simulink model "EulerPIDJoint_Copy"  (Simulink 7.6)
settings: Solver=ode3  StartTime=0.0  StopTime=8  FixedStep=Ts  RelTol=1e-3
InitFcn:
  | eval('Config');
  | eval('RobotCtlCfg');
values from neighbouring files (symbols this model uses):
  a2 = 0    [Config.m]    (also in CtrPlatformCfg.m)
  a3 = 0    [Config.m]    (also in CtrPlatformCfg.m)
  a4 = 0    [Config.m]    (also in CtrPlatformCfg.m)
  a5 = 90    [Config.m]    (also in CtrPlatformCfg.m)
  a6 = 0    [Config.m]    (also in CtrPlatformCfg.m)
  Cen_EU = Cen    [DynEulerTest.m]
  DH_EU = [266     300     0       0       1016     0      174 ... (first row only)    [DynEulerTest.m]
  freq = tvel/radius    (= 1)    [Config.m]    (also in CtrPlatformCfg.m)
  Ft_EU = [0;0;0;0;0;0]    [DynEulerTest.m]
  Gravity = 9.8    [Config.m]    (also in CtrPlatformCfg.m)
  Ie_EU = [Ie1;Ie2;Ie3;Ie4;Ie5;Ie6]    [DynEulerTest.m]
  in1 = [5.2954 -0.2565 -0.6366;-0.2565 4.7000 0.2830;-0.6366 0.2829 5.8635]    [Config.m]    (also in CtrPlatformCfg.m; DynEulerTest.m; EfDynCAD.m = [0.54  -0.01 0.23)
  in2 = [5.8840 0.0072 0.0135;0.0072 6.0178 -0.1907;0.0135 -0.1907 0.3374]    [Config.m]    (also in CtrPlatformCfg.m; DynEulerTest.m; EfDynCAD.m = (R_x*R_z)*in2*(R_x*R_z)')
  in3 = [1.8201 -0.2274 -0.3112;-0.2274 2.2537 -0.1441;-0.3112 -0.1441 1.9485]    [Config.m]    (also in CtrPlatformCfg.m; DynEulerTest.m; EfDynCAD.m = (R_x*R_z)*in3*(R_x*R_z)')
  in4 = [0.0607 -0.0922 0;-0.0922 1.4493 0;0 0 1.4620]    [Config.m]    (also in CtrPlatformCfg.m; DynEulerTest.m = [0.0607 -0.0922 0;-0.0922 1.4493 0;0 0,1.4620]; EfDynCAD.m = (R_y*Rz)*in4*(R_y*Rz)')
  in5 = [0.0191 0.0032 0;0.0032 0.0228 0;0 0 0.0291]    [Config.m]    (also in CtrPlatformCfg.m; DynEulerTest.m; EfDynCAD.m = (R_x*R_y)*in5*(R_x*R_y)')
  in6 = [0.0012 0 0;0 0.0007 0;0 0 0.0007]    [Config.m]    (also in CtrPlatformCfg.m; DynEulerTest.m; EfDynCAD.m = (R_y*Rz)*in6*(R_y*Rz)')
  init_Endx = gd_init(1,4)    [Config.m]    (also in CtrPlatformCfg.m)
  init_Endy = gd_init(2,4)    [Config.m]    (also in CtrPlatformCfg.m)
  init_Endz = gd_init(3,4)    [Config.m]    (also in CtrPlatformCfg.m)
  init_Rot = gd_init(1:3,1:3)    [Config.m]    (also in CtrPlatformCfg.m)
  L = [l1 l2 l3 l4 l5 l6 l7 l8 l9]    [Config.m]    (also in CtrPlatformCfg.m)
  ma1 = 170.31    [Config.m]    (also in CtrPlatformCfg.m; DynEulerTest.m; EfDynCAD.m = 77.75)
  ma2 = 63.74    [Config.m]    (also in CtrPlatformCfg.m; DynEulerTest.m; EfDynCAD.m = 32.31)
  ma3 = 98.98    [Config.m]    (also in CtrPlatformCfg.m; DynEulerTest.m; EfDynCAD.m = 18.61)
  ma4 = 24.46    [Config.m]    (also in CtrPlatformCfg.m; DynEulerTest.m; EfDynCAD.m = 15.65)
  ma5 = 5.24    [Config.m]    (also in CtrPlatformCfg.m; DynEulerTest.m; EfDynCAD.m = 3.32)
  ma6 = 0.6    [Config.m]    (also in CtrPlatformCfg.m; DynEulerTest.m; EfDynCAD.m)
  Ma_EU = Ma    [DynEulerTest.m]
  Rad2Line = Gear*EncRes/(2*pi)    [Config.m]    (also in CtrPlatformCfg.m)
  Ts = 1/FrHz    (= 0.00025)    [Config.m]    (also in CtrPlatformCfg.m)
  tvel = 120    [Config.m]    (also in CtrPlatformCfg.m)
undefined symbols (not defined in the file or in its folder): a1, DiscIntNeverNeededParam, jointAugKp, jointAugKv, PRBSGain, PRBSOffset, PRBSTimeLength, PulseFrq, PulseGain, RobotAxis, SineFrq, SineGain, V2T
libraries: simulink x58, mblibv1 x41, powerlib_extras x7
(part 4 of 5)

== system EulerPIDJoint_Copy/Display/GeneralAccDisplay/Jnt3/Display ==
  GeneralAcc3 : Inport
  Ref_GeneralAcc3 : Inport  Port=2
  AVx : Scope  NumInputPorts=2
      settings: TimeRange=10  YMin=-2.999999999999999e-017~-1  YMax=4e-017~1
  "AVy " : Scope  NumInputPorts=2
      settings: YMin=-5~-5  YMax=5~5
  AVz : Scope  NumInputPorts=2
      settings: YMin=-5~-5  YMax=5~5  SaveName=ScopeData2
  AWx : Scope  NumInputPorts=2
      settings: YMin=-5~-5  YMax=5~5  SaveName=ScopeData3
  AWy : Scope  NumInputPorts=2
      settings: TimeRange=10  YMin=-4.18~4.060000000000001  YMax=-4.04~4.2  SaveName=ScopeData4
  AWz : Scope  NumInputPorts=2
      settings: TimeRange=10  YMin=-1.6e-006~-0.003  YMax=4e-007~0.004  SaveName=ScopeData5
  Demux : Demux  Outputs=6
  Demux1 : Demux  Outputs=6
  "Encoder " : ToWorkspace  VariableName=EncGenAccJ3  SampleTime=-1  SaveFormat=Structure
  Err{1..6} (6 alike) : Scope
      Err1 settings: SaveName=ScopeData6
      Err2 settings: SaveName=ScopeData7
      Err3 settings: SaveName=ScopeData8
      Err4 settings: SaveName=ScopeData9
      Err5 settings: TimeRange=3  YMin=-2.5  YMax=1  SaveName=ScopeData10
      Err6 settings: SaveName=ScopeData11
  "Ref " : ToWorkspace  VariableName=RefGenAccJ3  SampleTime=-1  SaveFormat=Structure
  Sum{,1..5} (6 alike) : Sum  Inputs=+|-
  wires:
  Demux1/6 -> Sum5/2, AWz/2
  Demux1/5 -> Sum4/2, AWy/2
  Demux1/4 -> AWx/2, Sum3/2
  Demux1/3 -> Sum2/2, AVz/2
  Demux1/2 -> Sum1/2, "AVy "/2
  Demux/6 -> Sum5/1, AWz/1
  Demux/5 -> Sum4/1, AWy/1
  Demux/4 -> AWx/1, Sum3/1
  Demux/3 -> Sum2/1, AVz/1
  Demux/2 -> Sum1/1, "AVy "/1
  Demux1/1 -> AVx/2, Sum/2
  Demux/1 -> AVx/1, Sum/1
  Ref_GeneralAcc3/1 -> "Ref "/1, Demux1/1
  GeneralAcc3/1 -> "Encoder "/1, Demux/1
  Sum5/1 -> Err6/1
  Sum4/1 -> Err5/1
  Sum3/1 -> Err4/1
  Sum2/1 -> Err3/1
  Sum1/1 -> Err2/1
  Sum/1 -> Err1/1

== system EulerPIDJoint_Copy/Display/GeneralAccDisplay/Jnt4/Display ==
  GeneralAcc4 : Inport
  Ref_GeneralAcc4 : Inport  Port=2
  AVx : Scope  NumInputPorts=2
      settings: TimeRange=10  YMin=-2.999999999999999e-017~-1  YMax=4e-017~1
  "AVy " : Scope  NumInputPorts=2
      settings: YMin=-5~-5  YMax=5~5
  AVz : Scope  NumInputPorts=2
      settings: YMin=-5~-5  YMax=5~5  SaveName=ScopeData2
  AWx : Scope  NumInputPorts=2
      settings: YMin=-5~-5  YMax=5~5  SaveName=ScopeData3
  AWy : Scope  NumInputPorts=2
      settings: TimeRange=10  YMin=-4.18~4.060000000000001  YMax=-4.04~4.2  SaveName=ScopeData4
  AWz : Scope  NumInputPorts=2
      settings: TimeRange=10  YMin=-1.6e-006~-0.003  YMax=4e-007~0.004  SaveName=ScopeData5
  Demux : Demux  Outputs=6
  Demux1 : Demux  Outputs=6
  "Encoder " : ToWorkspace  VariableName=EncGenAccJ4  SampleTime=-1  SaveFormat=Structure
  Err{1..6} (6 alike) : Scope
      Err1 settings: SaveName=ScopeData6
      Err2 settings: SaveName=ScopeData7
      Err3 settings: SaveName=ScopeData8
      Err4 settings: SaveName=ScopeData9
      Err5 settings: TimeRange=3  YMin=-2.5  YMax=1  SaveName=ScopeData10
      Err6 settings: SaveName=ScopeData11
  "Ref " : ToWorkspace  VariableName=RefGenAccJ4  SampleTime=-1  SaveFormat=Structure
  Sum{,1..5} (6 alike) : Sum  Inputs=+|-
  wires:
  Sum/1 -> Err1/1
  Sum1/1 -> Err2/1
  Sum2/1 -> Err3/1
  Sum3/1 -> Err4/1
  Sum4/1 -> Err5/1
  Sum5/1 -> Err6/1
  GeneralAcc4/1 -> Demux/1, "Encoder "/1
  Ref_GeneralAcc4/1 -> Demux1/1, "Ref "/1
  Demux/1 -> Sum/1, AVx/1
  Demux1/1 -> Sum/2, AVx/2
  Demux/2 -> "AVy "/1, Sum1/1
  Demux/3 -> AVz/1, Sum2/1
  Demux/4 -> Sum3/1, AWx/1
  Demux/5 -> AWy/1, Sum4/1
  Demux/6 -> AWz/1, Sum5/1
  Demux1/2 -> "AVy "/2, Sum1/2
  Demux1/3 -> AVz/2, Sum2/2
  Demux1/4 -> Sum3/2, AWx/2
  Demux1/5 -> AWy/2, Sum4/2
  Demux1/6 -> AWz/2, Sum5/2

== system EulerPIDJoint_Copy/Display/GeneralAccDisplay/Jnt5/Display ==
  GeneralAcc5 : Inport
  Ref_GeneralAcc5 : Inport  Port=2
  AVx : Scope  NumInputPorts=2
      settings: TimeRange=10  YMin=-2.999999999999999e-017~-1  YMax=4e-017~1
  "AVy " : Scope  NumInputPorts=2
      settings: YMin=-5~-5  YMax=5~5
  AVz : Scope  NumInputPorts=2
      settings: YMin=-5~-5  YMax=5~5  SaveName=ScopeData2
  AWx : Scope  NumInputPorts=2
      settings: YMin=-5~-5  YMax=5~5  SaveName=ScopeData3
  AWy : Scope  NumInputPorts=2
      settings: TimeRange=10  YMin=-4.18~4.060000000000001  YMax=-4.04~4.2  SaveName=ScopeData4
  AWz : Scope  NumInputPorts=2
      settings: TimeRange=10  YMin=-1.6e-006~-0.003  YMax=4e-007~0.004  SaveName=ScopeData5
  Demux : Demux  Outputs=6
  Demux1 : Demux  Outputs=6
  "Encoder " : ToWorkspace  VariableName=EncGenAccJ5  SampleTime=-1  SaveFormat=Structure
  Err{1..6} (6 alike) : Scope
      Err1 settings: SaveName=ScopeData6
      Err2 settings: SaveName=ScopeData7
      Err3 settings: SaveName=ScopeData8
      Err4 settings: SaveName=ScopeData9
      Err5 settings: TimeRange=3  YMin=-2.5  YMax=1  SaveName=ScopeData10
      Err6 settings: SaveName=ScopeData11
  "Ref " : ToWorkspace  VariableName=RefGenAccJ5  SampleTime=-1  SaveFormat=Structure
  Sum{,1..5} (6 alike) : Sum  Inputs=+|-
  wires:
  Demux1/6 -> Sum5/2, AWz/2
  Demux1/5 -> Sum4/2, AWy/2
  Demux1/4 -> AWx/2, Sum3/2
  Demux1/3 -> Sum2/2, AVz/2
  Demux1/2 -> Sum1/2, "AVy "/2
  Demux/6 -> Sum5/1, AWz/1
  Demux/5 -> Sum4/1, AWy/1
  Demux/4 -> AWx/1, Sum3/1
  Demux/3 -> Sum2/1, AVz/1
  Demux/2 -> Sum1/1, "AVy "/1
  Demux1/1 -> AVx/2, Sum/2
  Demux/1 -> AVx/1, Sum/1
  Ref_GeneralAcc5/1 -> "Ref "/1, Demux1/1
  GeneralAcc5/1 -> "Encoder "/1, Demux/1
  Sum5/1 -> Err6/1
  Sum4/1 -> Err5/1
  Sum3/1 -> Err4/1
  Sum2/1 -> Err3/1
  Sum1/1 -> Err2/1
  Sum/1 -> Err1/1

== system EulerPIDJoint_Copy/Display/GeneralAccDisplay/Jnt6/Display ==
  GeneralAcc6 : Inport
  Ref_GeneralAcc6 : Inport  Port=2
  AVx : Scope  NumInputPorts=2
      settings: TimeRange=10  YMin=-2.999999999999999e-017~-1  YMax=4e-017~1
  "AVy " : Scope  NumInputPorts=2
      settings: YMin=-5~-5  YMax=5~5
  AVz : Scope  NumInputPorts=2
      settings: YMin=-5~-5  YMax=5~5  SaveName=ScopeData2
  AWx : Scope  NumInputPorts=2
      settings: YMin=-5~-5  YMax=5~5  SaveName=ScopeData3
  AWy : Scope  NumInputPorts=2
      settings: TimeRange=10  YMin=-4.18~4.060000000000001  YMax=-4.04~4.2  SaveName=ScopeData4
  AWz : Scope  NumInputPorts=2
      settings: TimeRange=10  YMin=-1.6e-006~-0.003  YMax=4e-007~0.004  SaveName=ScopeData5
  Demux : Demux  Outputs=6
  Demux1 : Demux  Outputs=6
  "Encoder " : ToWorkspace  VariableName=EncGenAccJ6  SampleTime=-1  SaveFormat=Structure
  Err{1..6} (6 alike) : Scope
      Err1 settings: SaveName=ScopeData6
      Err2 settings: SaveName=ScopeData7
      Err3 settings: SaveName=ScopeData8
      Err4 settings: SaveName=ScopeData9
      Err5 settings: TimeRange=3  YMin=-2.5  YMax=1  SaveName=ScopeData10
      Err6 settings: SaveName=ScopeData11
  "Ref " : ToWorkspace  VariableName=RefGenAccJ6  SampleTime=-1  SaveFormat=Structure
  Sum{,1..5} (6 alike) : Sum  Inputs=+|-
  wires:
  Sum/1 -> Err1/1
  Sum1/1 -> Err2/1
  Sum2/1 -> Err3/1
  Sum3/1 -> Err4/1
  Sum4/1 -> Err5/1
  Sum5/1 -> Err6/1
  GeneralAcc6/1 -> Demux/1, "Encoder "/1
  Ref_GeneralAcc6/1 -> Demux1/1, "Ref "/1
  Demux/1 -> Sum/1, AVx/1
  Demux1/1 -> Sum/2, AVx/2
  Demux/2 -> "AVy "/1, Sum1/1
  Demux/3 -> AVz/1, Sum2/1
  Demux/4 -> Sum3/1, AWx/1
  Demux/5 -> AWy/1, Sum4/1
  Demux/6 -> AWz/1, Sum5/1
  Demux1/2 -> "AVy "/2, Sum1/2
  Demux1/3 -> AVz/2, Sum2/2
  Demux1/4 -> Sum3/2, AWx/2
  Demux1/5 -> AWy/2, Sum4/2
  Demux1/6 -> AWz/2, Sum5/2

== system EulerPIDJoint_Copy/Display/GeneralForceDisplay/Jnt1/Display ==
  GeneralForce1 : Inport
  Ref_GeneralForce1 : Inport  Port=2
  Demux : Demux  Outputs=6
  Demux1 : Demux  Outputs=6
  "Encoder " : ToWorkspace  VariableName=EncGenForceJ1  SampleTime=-1  SaveFormat=Structure
  Err{1..6} (6 alike) : Scope
      Err1 settings: SaveName=ScopeData6
      Err2 settings: SaveName=ScopeData7
      Err3 settings: SaveName=ScopeData8
      Err4 settings: SaveName=ScopeData9
      Err5 settings: TimeRange=3  YMin=-2.5  YMax=1  SaveName=ScopeData10
      Err6 settings: SaveName=ScopeData11
  "Ref " : ToWorkspace  VariableName=RefGenForceJ1  SampleTime=-1  SaveFormat=Structure
  Sum{,1..5} (6 alike) : Sum  Inputs=+|-
  fx : Scope  NumInputPorts=2
      settings: TimeRange=10  YMin=-2.999999999999999e-017~-1  YMax=4e-017~1
  "fy " : Scope  NumInputPorts=2
      settings: YMin=-5~-5  YMax=5~5
  fz : Scope  NumInputPorts=2
      settings: YMin=-5~-5  YMax=5~5  SaveName=ScopeData2
  taux : Scope  NumInputPorts=2
      settings: YMin=-5~-5  YMax=5~5  SaveName=ScopeData3
  tauy : Scope  NumInputPorts=2
      settings: TimeRange=10  YMin=-4.18~4.060000000000001  YMax=-4.04~4.2  SaveName=ScopeData4
  tauz : Scope  NumInputPorts=2
      settings: TimeRange=10  YMin=-1.6e-006~-0.003  YMax=4e-007~0.004  SaveName=ScopeData5
  wires:
  Sum/1 -> Err1/1
  Sum1/1 -> Err2/1
  Sum2/1 -> Err3/1
  Sum3/1 -> Err4/1
  Sum4/1 -> Err5/1
  Sum5/1 -> Err6/1
  GeneralForce1/1 -> Demux/1, "Encoder "/1
  Ref_GeneralForce1/1 -> Demux1/1, "Ref "/1
  Demux/1 -> Sum/1, fx/1
  Demux1/1 -> Sum/2, fx/2
  Demux/2 -> "fy "/1, Sum1/1
  Demux/3 -> fz/1, Sum2/1
  Demux/4 -> Sum3/1, taux/1
  Demux/5 -> tauy/1, Sum4/1
  Demux/6 -> tauz/1, Sum5/1
  Demux1/2 -> "fy "/2, Sum1/2
  Demux1/3 -> fz/2, Sum2/2
  Demux1/4 -> Sum3/2, taux/2
  Demux1/5 -> tauy/2, Sum4/2
  Demux1/6 -> tauz/2, Sum5/2

== system EulerPIDJoint_Copy/Display/GeneralForceDisplay/Jnt2/Display ==
  GeneralForce2 : Inport
  Ref_GeneralForce2 : Inport  Port=2
  Demux : Demux  Outputs=6
  Demux1 : Demux  Outputs=6
  "Encoder " : ToWorkspace  VariableName=EncGenForceJ2  SampleTime=-1  SaveFormat=Structure
  Err{1..6} (6 alike) : Scope
      Err1 settings: SaveName=ScopeData6
      Err2 settings: SaveName=ScopeData7
      Err3 settings: SaveName=ScopeData8
      Err4 settings: SaveName=ScopeData9
      Err5 settings: TimeRange=3  YMin=-2.5  YMax=1  SaveName=ScopeData10
      Err6 settings: SaveName=ScopeData11
  "Ref " : ToWorkspace  VariableName=RefGenForceJ2  SampleTime=-1  SaveFormat=Structure
  Sum{,1..5} (6 alike) : Sum  Inputs=+|-
  fx : Scope  NumInputPorts=2
      settings: TimeRange=10  YMin=-2.999999999999999e-017~-1  YMax=4e-017~1
  "fy " : Scope  NumInputPorts=2
      settings: YMin=-5~-5  YMax=5~5
  fz : Scope  NumInputPorts=2
      settings: YMin=-5~-5  YMax=5~5  SaveName=ScopeData2
  taux : Scope  NumInputPorts=2
      settings: YMin=-5~-5  YMax=5~5  SaveName=ScopeData3
  tauy : Scope  NumInputPorts=2
      settings: TimeRange=10  YMin=-4.18~4.060000000000001  YMax=-4.04~4.2  SaveName=ScopeData4
  tauz : Scope  NumInputPorts=2
      settings: TimeRange=10  YMin=-1.6e-006~-0.003  YMax=4e-007~0.004  SaveName=ScopeData5
  wires:
  Sum/1 -> Err1/1
  Sum1/1 -> Err2/1
  Sum2/1 -> Err3/1
  Sum3/1 -> Err4/1
  Sum4/1 -> Err5/1
  Sum5/1 -> Err6/1
  GeneralForce2/1 -> Demux/1, "Encoder "/1
  Ref_GeneralForce2/1 -> Demux1/1, "Ref "/1
  Demux/1 -> Sum/1, fx/1
  Demux1/1 -> Sum/2, fx/2
  Demux/2 -> "fy "/1, Sum1/1
  Demux/3 -> fz/1, Sum2/1
  Demux/4 -> Sum3/1, taux/1
  Demux/5 -> tauy/1, Sum4/1
  Demux/6 -> tauz/1, Sum5/1
  Demux1/2 -> "fy "/2, Sum1/2
  Demux1/3 -> fz/2, Sum2/2
  Demux1/4 -> Sum3/2, taux/2
  Demux1/5 -> tauy/2, Sum4/2
  Demux1/6 -> tauz/2, Sum5/2

== system EulerPIDJoint_Copy/Display/GeneralForceDisplay/Jnt3/Display ==
  GeneralForce3 : Inport
  Ref_GeneralForce3 : Inport  Port=2
  Demux : Demux  Outputs=6
  Demux1 : Demux  Outputs=6
  "Encoder " : ToWorkspace  VariableName=EncGenForceJ3  SampleTime=-1  SaveFormat=Structure
  Err{1..6} (6 alike) : Scope
      Err1 settings: SaveName=ScopeData6
      Err2 settings: SaveName=ScopeData7
      Err3 settings: SaveName=ScopeData8
      Err4 settings: SaveName=ScopeData9
      Err5 settings: TimeRange=3  YMin=-2.5  YMax=1  SaveName=ScopeData10
      Err6 settings: SaveName=ScopeData11
  "Ref " : ToWorkspace  VariableName=RefGenForceJ3  SampleTime=-1  SaveFormat=Structure
  Sum{,1..5} (6 alike) : Sum  Inputs=+|-
  fx : Scope  NumInputPorts=2
      settings: TimeRange=10  YMin=-2.999999999999999e-017~-1  YMax=4e-017~1
  "fy " : Scope  NumInputPorts=2
      settings: YMin=-5~-5  YMax=5~5
  fz : Scope  NumInputPorts=2
      settings: YMin=-5~-5  YMax=5~5  SaveName=ScopeData2
  taux : Scope  NumInputPorts=2
      settings: YMin=-5~-5  YMax=5~5  SaveName=ScopeData3
  tauy : Scope  NumInputPorts=2
      settings: TimeRange=10  YMin=-4.18~4.060000000000001  YMax=-4.04~4.2  SaveName=ScopeData4
  tauz : Scope  NumInputPorts=2
      settings: TimeRange=10  YMin=-1.6e-006~-0.003  YMax=4e-007~0.004  SaveName=ScopeData5
  wires:
  Sum/1 -> Err1/1
  Sum1/1 -> Err2/1
  Sum2/1 -> Err3/1
  Sum3/1 -> Err4/1
  Sum4/1 -> Err5/1
  Sum5/1 -> Err6/1
  GeneralForce3/1 -> Demux/1, "Encoder "/1
  Ref_GeneralForce3/1 -> Demux1/1, "Ref "/1
  Demux/1 -> Sum/1, fx/1
  Demux1/1 -> Sum/2, fx/2
  Demux/2 -> "fy "/1, Sum1/1
  Demux/3 -> fz/1, Sum2/1
  Demux/4 -> Sum3/1, taux/1
  Demux/5 -> tauy/1, Sum4/1
  Demux/6 -> tauz/1, Sum5/1
  Demux1/2 -> "fy "/2, Sum1/2
  Demux1/3 -> fz/2, Sum2/2
  Demux1/4 -> Sum3/2, taux/2
  Demux1/5 -> tauy/2, Sum4/2
  Demux1/6 -> tauz/2, Sum5/2

== system EulerPIDJoint_Copy/Display/GeneralForceDisplay/Jnt4/Display ==
  GeneralForce4 : Inport
  Ref_GeneralForce4 : Inport  Port=2
  Demux : Demux  Outputs=6
  Demux1 : Demux  Outputs=6
  "Encoder " : ToWorkspace  VariableName=EncGenForceJ4  SampleTime=-1  SaveFormat=Structure
  Err{1..6} (6 alike) : Scope
      Err1 settings: SaveName=ScopeData6
      Err2 settings: SaveName=ScopeData7
      Err3 settings: SaveName=ScopeData8
      Err4 settings: SaveName=ScopeData9
      Err5 settings: TimeRange=3  YMin=-2.5  YMax=1  SaveName=ScopeData10
      Err6 settings: SaveName=ScopeData11
  "Ref " : ToWorkspace  VariableName=RefGenForceJ4  SampleTime=-1  SaveFormat=Structure
  Sum{,1..5} (6 alike) : Sum  Inputs=+|-
  fx : Scope  NumInputPorts=2
      settings: TimeRange=10  YMin=-2.999999999999999e-017~-1  YMax=4e-017~1
  "fy " : Scope  NumInputPorts=2
      settings: YMin=-5~-5  YMax=5~5
  fz : Scope  NumInputPorts=2
      settings: YMin=-5~-5  YMax=5~5  SaveName=ScopeData2
  taux : Scope  NumInputPorts=2
      settings: YMin=-5~-5  YMax=5~5  SaveName=ScopeData3
  tauy : Scope  NumInputPorts=2
      settings: TimeRange=10  YMin=-4.18~4.060000000000001  YMax=-4.04~4.2  SaveName=ScopeData4
  tauz : Scope  NumInputPorts=2
      settings: TimeRange=10  YMin=-1.6e-006~-0.003  YMax=4e-007~0.004  SaveName=ScopeData5
  wires:
  Sum/1 -> Err1/1
  Sum1/1 -> Err2/1
  Sum2/1 -> Err3/1
  Sum3/1 -> Err4/1
  Sum4/1 -> Err5/1
  Sum5/1 -> Err6/1
  GeneralForce4/1 -> Demux/1, "Encoder "/1
  Ref_GeneralForce4/1 -> Demux1/1, "Ref "/1
  Demux/1 -> Sum/1, fx/1
  Demux1/1 -> Sum/2, fx/2
  Demux/2 -> "fy "/1, Sum1/1
  Demux/3 -> fz/1, Sum2/1
  Demux/4 -> Sum3/1, taux/1
  Demux/5 -> tauy/1, Sum4/1
  Demux/6 -> tauz/1, Sum5/1
  Demux1/2 -> "fy "/2, Sum1/2
  Demux1/3 -> fz/2, Sum2/2
  Demux1/4 -> Sum3/2, taux/2
  Demux1/5 -> tauy/2, Sum4/2
  Demux1/6 -> tauz/2, Sum5/2

== system EulerPIDJoint_Copy/Display/GeneralForceDisplay/Jnt5/Display ==
  GeneralForce5 : Inport
  Ref_GeneralForce5 : Inport  Port=2
  Demux : Demux  Outputs=6
  Demux1 : Demux  Outputs=6
  "Encoder " : ToWorkspace  VariableName=EncGenForceJ5  SampleTime=-1  SaveFormat=Structure
  Err{1..6} (6 alike) : Scope
      Err1 settings: SaveName=ScopeData6
      Err2 settings: SaveName=ScopeData7
      Err3 settings: SaveName=ScopeData8
      Err4 settings: SaveName=ScopeData9
      Err5 settings: TimeRange=3  YMin=-2.5  YMax=1  SaveName=ScopeData10
      Err6 settings: SaveName=ScopeData11
  "Ref " : ToWorkspace  VariableName=RefGenForceJ5  SampleTime=-1  SaveFormat=Structure
  Sum{,1..5} (6 alike) : Sum  Inputs=+|-
  fx : Scope  NumInputPorts=2
      settings: TimeRange=10  YMin=-2.999999999999999e-017~-1  YMax=4e-017~1
  "fy " : Scope  NumInputPorts=2
      settings: YMin=-5~-5  YMax=5~5
  fz : Scope  NumInputPorts=2
      settings: YMin=-5~-5  YMax=5~5  SaveName=ScopeData2
  taux : Scope  NumInputPorts=2
      settings: YMin=-5~-5  YMax=5~5  SaveName=ScopeData3
  tauy : Scope  NumInputPorts=2
      settings: TimeRange=10  YMin=-4.18~4.060000000000001  YMax=-4.04~4.2  SaveName=ScopeData4
  tauz : Scope  NumInputPorts=2
      settings: TimeRange=10  YMin=-1.6e-006~-0.003  YMax=4e-007~0.004  SaveName=ScopeData5
  wires:
  Sum/1 -> Err1/1
  Sum1/1 -> Err2/1
  Sum2/1 -> Err3/1
  Sum3/1 -> Err4/1
  Sum4/1 -> Err5/1
  Sum5/1 -> Err6/1
  GeneralForce5/1 -> Demux/1, "Encoder "/1
  Ref_GeneralForce5/1 -> Demux1/1, "Ref "/1
  Demux/1 -> Sum/1, fx/1
  Demux1/1 -> Sum/2, fx/2
  Demux/2 -> "fy "/1, Sum1/1
  Demux/3 -> fz/1, Sum2/1
  Demux/4 -> Sum3/1, taux/1
  Demux/5 -> tauy/1, Sum4/1
  Demux/6 -> tauz/1, Sum5/1
  Demux1/2 -> "fy "/2, Sum1/2
  Demux1/3 -> fz/2, Sum2/2
  Demux1/4 -> Sum3/2, taux/2
  Demux1/5 -> tauy/2, Sum4/2
  Demux1/6 -> tauz/2, Sum5/2

== system EulerPIDJoint_Copy/Display/GeneralForceDisplay/Jnt6/Display ==
  GeneralForce6 : Inport
  Ref_GeneralForce6 : Inport  Port=2
  Demux : Demux  Outputs=6
  Demux1 : Demux  Outputs=6
  "Encoder " : ToWorkspace  VariableName=EncGenForceJ6  SampleTime=-1  SaveFormat=Structure
  Err{1..6} (6 alike) : Scope
      Err1 settings: SaveName=ScopeData6
      Err2 settings: SaveName=ScopeData7
      Err3 settings: SaveName=ScopeData8
      Err4 settings: SaveName=ScopeData9
      Err5 settings: TimeRange=3  YMin=-2.5  YMax=1  SaveName=ScopeData10
      Err6 settings: SaveName=ScopeData11
  "Ref " : ToWorkspace  VariableName=RefGenForceJ6  SampleTime=-1  SaveFormat=Structure
  Sum{,1..5} (6 alike) : Sum  Inputs=+|-
  fx : Scope  NumInputPorts=2
      settings: TimeRange=10  YMin=-2.999999999999999e-017~-1  YMax=4e-017~1
  "fy " : Scope  NumInputPorts=2
      settings: YMin=-5~-5  YMax=5~5
  fz : Scope  NumInputPorts=2
      settings: YMin=-5~-5  YMax=5~5  SaveName=ScopeData2
  taux : Scope  NumInputPorts=2
      settings: YMin=-5~-5  YMax=5~5  SaveName=ScopeData3
  tauy : Scope  NumInputPorts=2
      settings: TimeRange=10  YMin=-4.18~4.060000000000001  YMax=-4.04~4.2  SaveName=ScopeData4
  tauz : Scope  NumInputPorts=2
      settings: TimeRange=10  YMin=-1.6e-006~-0.003  YMax=4e-007~0.004  SaveName=ScopeData5
  wires:
  Sum/1 -> Err1/1
  Sum1/1 -> Err2/1
  Sum2/1 -> Err3/1
  Sum3/1 -> Err4/1
  Sum4/1 -> Err5/1
  Sum5/1 -> Err6/1
  GeneralForce6/1 -> Demux/1, "Encoder "/1
  Ref_GeneralForce6/1 -> Demux1/1, "Ref "/1
  Demux/1 -> Sum/1, fx/1
  Demux1/1 -> Sum/2, fx/2
  Demux/2 -> "fy "/1, Sum1/1
  Demux/3 -> fz/1, Sum2/1
  Demux/4 -> Sum3/1, taux/1
  Demux/5 -> tauy/1, Sum4/1
  Demux/6 -> tauz/1, Sum5/1
  Demux1/2 -> "fy "/2, Sum1/2
  Demux1/3 -> fz/2, Sum2/2
  Demux1/4 -> Sum3/2, taux/2
  Demux1/5 -> tauy/2, Sum4/2
  Demux1/6 -> tauz/2, Sum5/2

== system EulerPIDJoint_Copy/Display/GeneralVelDisplay/Jnt1/Display ==
  GeneralVel1 : Inport
  Ref_GeneralVel1 : Inport  Port=2
  Demux : Demux  Outputs=6
  Demux1 : Demux  Outputs=6
  "Encoder " : ToWorkspace  VariableName=EncGenVelJ1  SampleTime=-1  SaveFormat=Structure
  Err{1..6} (6 alike) : Scope
      Err1 settings: SaveName=ScopeData6
      Err2 settings: SaveName=ScopeData7
      Err3 settings: SaveName=ScopeData8
      Err4 settings: SaveName=ScopeData9
      Err5 settings: TimeRange=3  YMin=-2.5  YMax=1  SaveName=ScopeData10
      Err6 settings: SaveName=ScopeData11
  "Ref " : ToWorkspace  VariableName=RefGenVelJ1  SampleTime=-1  SaveFormat=Structure
  Sum{,1..5} (6 alike) : Sum  Inputs=+|-
  Vx : Scope  NumInputPorts=2
      settings: TimeRange=10  YMin=-2.999999999999999e-017~-1  YMax=4e-017~1
  "Vy " : Scope  NumInputPorts=2
      settings: YMin=-5~-5  YMax=5~5
  Vz : Scope  NumInputPorts=2
      settings: YMin=-5~-5  YMax=5~5  SaveName=ScopeData2
  Wx : Scope  NumInputPorts=2
      settings: YMin=-5~-5  YMax=5~5  SaveName=ScopeData3
  Wy : Scope  NumInputPorts=2
      settings: TimeRange=10  YMin=-4.18~4.060000000000001  YMax=-4.04~4.2  SaveName=ScopeData4
  Wz : Scope  NumInputPorts=2
      settings: TimeRange=10  YMin=-1.6e-006~-0.003  YMax=4e-007~0.004  SaveName=ScopeData5
  wires:
  Sum/1 -> Err1/1
  Sum1/1 -> Err2/1
  Sum2/1 -> Err3/1
  Sum3/1 -> Err4/1
  Sum4/1 -> Err5/1
  Sum5/1 -> Err6/1
  GeneralVel1/1 -> Demux/1, "Encoder "/1
  Ref_GeneralVel1/1 -> Demux1/1, "Ref "/1
  Demux/1 -> Sum/1, Vx/1
  Demux1/1 -> Sum/2, Vx/2
  Demux/2 -> "Vy "/1, Sum1/1
  Demux/3 -> Vz/1, Sum2/1
  Demux/4 -> Sum3/1, Wx/1
  Demux/5 -> Wy/1, Sum4/1
  Demux/6 -> Wz/1, Sum5/1
  Demux1/2 -> "Vy "/2, Sum1/2
  Demux1/3 -> Vz/2, Sum2/2
  Demux1/4 -> Sum3/2, Wx/2
  Demux1/5 -> Wy/2, Sum4/2
  Demux1/6 -> Wz/2, Sum5/2

== system EulerPIDJoint_Copy/Display/GeneralVelDisplay/Jnt2/Display ==
  GeneralVel2 : Inport
  Ref_GeneralVel2 : Inport  Port=2
  Demux : Demux  Outputs=6
  Demux1 : Demux  Outputs=6
  "Encoder " : ToWorkspace  VariableName=EncGenVelJ2  SampleTime=-1  SaveFormat=Structure
  Err{1..6} (6 alike) : Scope
      Err1 settings: SaveName=ScopeData6
      Err2 settings: SaveName=ScopeData7
      Err3 settings: SaveName=ScopeData8
      Err4 settings: SaveName=ScopeData9
      Err5 settings: TimeRange=3  YMin=-2.5  YMax=1  SaveName=ScopeData10
      Err6 settings: SaveName=ScopeData11
  "Ref " : ToWorkspace  VariableName=RefGenVelJ2  SampleTime=-1  SaveFormat=Structure
  Sum{,1..5} (6 alike) : Sum  Inputs=+|-
  Vx : Scope  NumInputPorts=2
      settings: TimeRange=10  YMin=-2.999999999999999e-017~-1  YMax=4e-017~1
  "Vy " : Scope  NumInputPorts=2
      settings: YMin=-5~-5  YMax=5~5
  Vz : Scope  NumInputPorts=2
      settings: YMin=-5~-5  YMax=5~5  SaveName=ScopeData2
  Wx : Scope  NumInputPorts=2
      settings: YMin=-5~-5  YMax=5~5  SaveName=ScopeData3
  Wy : Scope  NumInputPorts=2
      settings: TimeRange=10  YMin=-4.18~4.060000000000001  YMax=-4.04~4.2  SaveName=ScopeData4
  Wz : Scope  NumInputPorts=2
      settings: TimeRange=10  YMin=-1.6e-006~-0.003  YMax=4e-007~0.004  SaveName=ScopeData5
  wires:
  Demux1/6 -> Sum5/2, Wz/2
  Demux1/5 -> Sum4/2, Wy/2
  Demux1/4 -> Wx/2, Sum3/2
  Demux1/3 -> Sum2/2, Vz/2
  Demux1/2 -> Sum1/2, "Vy "/2
  Demux/6 -> Sum5/1, Wz/1
  Demux/5 -> Sum4/1, Wy/1
  Demux/4 -> Wx/1, Sum3/1
  Demux/3 -> Sum2/1, Vz/1
  Demux/2 -> Sum1/1, "Vy "/1
  Demux1/1 -> Vx/2, Sum/2
  Demux/1 -> Vx/1, Sum/1
  Ref_GeneralVel2/1 -> "Ref "/1, Demux1/1
  GeneralVel2/1 -> "Encoder "/1, Demux/1
  Sum5/1 -> Err6/1
  Sum4/1 -> Err5/1
  Sum3/1 -> Err4/1
  Sum2/1 -> Err3/1
  Sum1/1 -> Err2/1
  Sum/1 -> Err1/1

== system EulerPIDJoint_Copy/Display/GeneralVelDisplay/Jnt3/Display ==
  GeneralVel3 : Inport
  Ref_GeneralVel3 : Inport  Port=2
  Demux : Demux  Outputs=6
  Demux1 : Demux  Outputs=6
  "Encoder " : ToWorkspace  VariableName=EncGenVelJ3  SampleTime=-1  SaveFormat=Structure
  Err{1..6} (6 alike) : Scope
      Err1 settings: SaveName=ScopeData6
      Err2 settings: SaveName=ScopeData7
      Err3 settings: SaveName=ScopeData8
      Err4 settings: SaveName=ScopeData9
      Err5 settings: TimeRange=3  YMin=-2.5  YMax=1  SaveName=ScopeData10
      Err6 settings: SaveName=ScopeData11
  "Ref " : ToWorkspace  VariableName=RefGenVelJ3  SampleTime=-1  SaveFormat=Structure
  Sum{,1..5} (6 alike) : Sum  Inputs=+|-
  Vx : Scope  NumInputPorts=2
      settings: TimeRange=10  YMin=-2.999999999999999e-017~-1  YMax=4e-017~1
  "Vy " : Scope  NumInputPorts=2
      settings: YMin=-5~-5  YMax=5~5
  Vz : Scope  NumInputPorts=2
      settings: YMin=-5~-5  YMax=5~5  SaveName=ScopeData2
  Wx : Scope  NumInputPorts=2
      settings: YMin=-5~-5  YMax=5~5  SaveName=ScopeData3
  Wy : Scope  NumInputPorts=2
      settings: TimeRange=10  YMin=-4.18~4.060000000000001  YMax=-4.04~4.2  SaveName=ScopeData4
  Wz : Scope  NumInputPorts=2
      settings: TimeRange=10  YMin=-1.6e-006~-0.003  YMax=4e-007~0.004  SaveName=ScopeData5
  wires:
  Sum/1 -> Err1/1
  Sum1/1 -> Err2/1
  Sum2/1 -> Err3/1
  Sum3/1 -> Err4/1
  Sum4/1 -> Err5/1
  Sum5/1 -> Err6/1
  GeneralVel3/1 -> Demux/1, "Encoder "/1
  Ref_GeneralVel3/1 -> Demux1/1, "Ref "/1
  Demux/1 -> Sum/1, Vx/1
  Demux1/1 -> Sum/2, Vx/2
  Demux/2 -> "Vy "/1, Sum1/1
  Demux/3 -> Vz/1, Sum2/1
  Demux/4 -> Sum3/1, Wx/1
  Demux/5 -> Wy/1, Sum4/1
  Demux/6 -> Wz/1, Sum5/1
  Demux1/2 -> "Vy "/2, Sum1/2
  Demux1/3 -> Vz/2, Sum2/2
  Demux1/4 -> Sum3/2, Wx/2
  Demux1/5 -> Wy/2, Sum4/2
  Demux1/6 -> Wz/2, Sum5/2

== system EulerPIDJoint_Copy/Display/GeneralVelDisplay/Jnt4/Display ==
  GeneralVel4 : Inport
  Ref_GeneralVel4 : Inport  Port=2
  Demux : Demux  Outputs=6
  Demux1 : Demux  Outputs=6
  "Encoder " : ToWorkspace  VariableName=EncGenVelJ4  SampleTime=-1  SaveFormat=Structure
  Err{1..6} (6 alike) : Scope
      Err1 settings: SaveName=ScopeData6
      Err2 settings: SaveName=ScopeData7
      Err3 settings: SaveName=ScopeData8
      Err4 settings: SaveName=ScopeData9
      Err5 settings: TimeRange=3  YMin=-2.5  YMax=1  SaveName=ScopeData10
      Err6 settings: SaveName=ScopeData11
  "Ref " : ToWorkspace  VariableName=RefGenVelJ4  SampleTime=-1  SaveFormat=Structure
  Sum{,1..5} (6 alike) : Sum  Inputs=+|-
  Vx : Scope  NumInputPorts=2
      settings: TimeRange=10  YMin=-2.999999999999999e-017~-1  YMax=4e-017~1
  "Vy " : Scope  NumInputPorts=2
      settings: YMin=-5~-5  YMax=5~5
  Vz : Scope  NumInputPorts=2
      settings: YMin=-5~-5  YMax=5~5  SaveName=ScopeData2
  Wx : Scope  NumInputPorts=2
      settings: YMin=-5~-5  YMax=5~5  SaveName=ScopeData3
  Wy : Scope  NumInputPorts=2
      settings: TimeRange=10  YMin=-4.18~4.060000000000001  YMax=-4.04~4.2  SaveName=ScopeData4
  Wz : Scope  NumInputPorts=2
      settings: TimeRange=10  YMin=-1.6e-006~-0.003  YMax=4e-007~0.004  SaveName=ScopeData5
  wires:
  Demux1/6 -> Sum5/2, Wz/2
  Demux1/5 -> Sum4/2, Wy/2
  Demux1/4 -> Wx/2, Sum3/2
  Demux1/3 -> Sum2/2, Vz/2
  Demux1/2 -> Sum1/2, "Vy "/2
  Demux/6 -> Sum5/1, Wz/1
  Demux/5 -> Sum4/1, Wy/1
  Demux/4 -> Wx/1, Sum3/1
  Demux/3 -> Sum2/1, Vz/1
  Demux/2 -> Sum1/1, "Vy "/1
  Demux1/1 -> Vx/2, Sum/2
  Demux/1 -> Vx/1, Sum/1
  Ref_GeneralVel4/1 -> "Ref "/1, Demux1/1
  GeneralVel4/1 -> "Encoder "/1, Demux/1
  Sum5/1 -> Err6/1
  Sum4/1 -> Err5/1
  Sum3/1 -> Err4/1
  Sum2/1 -> Err3/1
  Sum1/1 -> Err2/1
  Sum/1 -> Err1/1

== system EulerPIDJoint_Copy/Display/GeneralVelDisplay/Jnt5/Display ==
  GeneralVel5 : Inport
  Ref_GeneralVel5 : Inport  Port=2
  Demux : Demux  Outputs=6
  Demux1 : Demux  Outputs=6
  "Encoder " : ToWorkspace  VariableName=EncGenVelJ5  SampleTime=-1  SaveFormat=Structure
  Err{1..6} (6 alike) : Scope
      Err1 settings: SaveName=ScopeData6
      Err2 settings: SaveName=ScopeData7
      Err3 settings: SaveName=ScopeData8
      Err4 settings: SaveName=ScopeData9
      Err5 settings: TimeRange=3  YMin=-2.5  YMax=1  SaveName=ScopeData10
      Err6 settings: SaveName=ScopeData11
  "Ref " : ToWorkspace  VariableName=RefGenVelJ5  SampleTime=-1  SaveFormat=Structure
  Sum{,1..5} (6 alike) : Sum  Inputs=+|-
  Vx : Scope  NumInputPorts=2
      settings: TimeRange=10  YMin=-2.999999999999999e-017~-1  YMax=4e-017~1
  "Vy " : Scope  NumInputPorts=2
      settings: YMin=-5~-5  YMax=5~5
  Vz : Scope  NumInputPorts=2
      settings: YMin=-5~-5  YMax=5~5  SaveName=ScopeData2
  Wx : Scope  NumInputPorts=2
      settings: YMin=-5~-5  YMax=5~5  SaveName=ScopeData3
  Wy : Scope  NumInputPorts=2
      settings: TimeRange=10  YMin=-4.18~4.060000000000001  YMax=-4.04~4.2  SaveName=ScopeData4
  Wz : Scope  NumInputPorts=2
      settings: TimeRange=10  YMin=-1.6e-006~-0.003  YMax=4e-007~0.004  SaveName=ScopeData5
  wires:
  Sum/1 -> Err1/1
  Sum1/1 -> Err2/1
  Sum2/1 -> Err3/1
  Sum3/1 -> Err4/1
  Sum4/1 -> Err5/1
  Sum5/1 -> Err6/1
  GeneralVel5/1 -> Demux/1, "Encoder "/1
  Ref_GeneralVel5/1 -> Demux1/1, "Ref "/1
  Demux/1 -> Sum/1, Vx/1
  Demux1/1 -> Sum/2, Vx/2
  Demux/2 -> "Vy "/1, Sum1/1
  Demux/3 -> Vz/1, Sum2/1
  Demux/4 -> Sum3/1, Wx/1
  Demux/5 -> Wy/1, Sum4/1
  Demux/6 -> Wz/1, Sum5/1
  Demux1/2 -> "Vy "/2, Sum1/2
  Demux1/3 -> Vz/2, Sum2/2
  Demux1/4 -> Sum3/2, Wx/2
  Demux1/5 -> Wy/2, Sum4/2
  Demux1/6 -> Wz/2, Sum5/2

== system EulerPIDJoint_Copy/Display/GeneralVelDisplay/Jnt6/Display ==
  GeneralVel6 : Inport
  Ref_GeneralVel6 : Inport  Port=2
  Demux : Demux  Outputs=6
  Demux1 : Demux  Outputs=6
  "Encoder " : ToWorkspace  VariableName=EncGenVelJ6  SampleTime=-1  SaveFormat=Structure
  Err{1..6} (6 alike) : Scope
      Err1 settings: SaveName=ScopeData6
      Err2 settings: SaveName=ScopeData7
      Err3 settings: SaveName=ScopeData8
      Err4 settings: SaveName=ScopeData9
      Err5 settings: TimeRange=3  YMin=-2.5  YMax=1  SaveName=ScopeData10
      Err6 settings: SaveName=ScopeData11
  "Ref " : ToWorkspace  VariableName=RefGenVelJ6  SampleTime=-1  SaveFormat=Structure
  Sum{,1..5} (6 alike) : Sum  Inputs=+|-
  Vx : Scope  NumInputPorts=2
      settings: TimeRange=10  YMin=-2.999999999999999e-017~-1  YMax=4e-017~1
  "Vy " : Scope  NumInputPorts=2
      settings: YMin=-5~-5  YMax=5~5
  Vz : Scope  NumInputPorts=2
      settings: YMin=-5~-5  YMax=5~5  SaveName=ScopeData2
  Wx : Scope  NumInputPorts=2
      settings: YMin=-5~-5  YMax=5~5  SaveName=ScopeData3
  Wy : Scope  NumInputPorts=2
      settings: TimeRange=10  YMin=-4.18~4.060000000000001  YMax=-4.04~4.2  SaveName=ScopeData4
  Wz : Scope  NumInputPorts=2
      settings: TimeRange=10  YMin=-1.6e-006~-0.003  YMax=4e-007~0.004  SaveName=ScopeData5
  wires:
  Demux1/6 -> Sum5/2, Wz/2
  Demux1/5 -> Sum4/2, Wy/2
  Demux1/4 -> Wx/2, Sum3/2
  Demux1/3 -> Sum2/2, Vz/2
  Demux1/2 -> Sum1/2, "Vy "/2
  Demux/6 -> Sum5/1, Wz/1
  Demux/5 -> Sum4/1, Wy/1
  Demux/4 -> Wx/1, Sum3/1
  Demux/3 -> Sum2/1, Vz/1
  Demux/2 -> Sum1/1, "Vy "/1
  Demux1/1 -> Vx/2, Sum/2
  Demux/1 -> Vx/1, Sum/1
  Ref_GeneralVel6/1 -> "Ref "/1, Demux1/1
  GeneralVel6/1 -> "Encoder "/1, Demux/1
  Sum5/1 -> Err6/1
  Sum4/1 -> Err5/1
  Sum3/1 -> Err4/1
  Sum2/1 -> Err3/1
  Sum1/1 -> Err2/1
  Sum/1 -> Err1/1

== system EulerPIDJoint_Copy/Controller/PID Controller/PID Controller/Controller Axis 1/EncDiff2Vel ==
  Enc : Inport
  Add : Sum  Inputs=+-
  Discrete  2nd-Order Filter : powerlib_extras/Discrete  Control Blocks/Discrete  2nd-Order Filter  DialogController=POWERSYS.PowerSysDialog  SystemSampleTime=-1  FilterType=Lowpass  Fo=1000  Zeta=0.707  Ts=Ts  Initialize=off  Vac_Init=[0.8 -25 60]  Vdc_Init=-0.4  PlotResponse=off  param1=[1 5000 10]
  Integer Delay : simulink/Discrete/Integer Delay  NumDelays=1  InputProcessing=Inherited  vinit=a1/180*pi  samptime=-1
  Vel : Outport
  wires:
  Add/1 -> Discrete  2nd-Order Filter/1
  Discrete  2nd-Order Filter/1 -> Vel/1
  Enc/1 -> Integer Delay/1, Add/1
  Integer Delay/1 -> Add/2

== system EulerPIDJoint_Copy/Controller/PID Controller/PID Controller/Controller Axis 1/Error Check and Lock Error ==
  CurrentCheck : Inport
  VelocityCheck : Inport  Port=2
  Abs : Abs
  Abs1 : Abs
  Compare To Constant : simulink/Logic and Bit Operations/Compare To Constant  SystemSampleTime=-1  relop=<=  const=VelErrorCheckLimit  LogicOutDataTypeMode=uint8  ZeroCross=off
  Compare To Constant1 : simulink/Logic and Bit Operations/Compare To Constant  SystemSampleTime=-1  relop=<=  const=VLLimit *1.01  LogicOutDataTypeMode=uint8  ZeroCross=off
  Logical Operator : Logic  Inputs=3  AllPortsSameDT=off  OutDataTypeStr=boolean
  Unit Delay : UnitDelay  X0=1  SampleTime=Ts
  ErrorFlag : Outport
  wires:
  VelocityCheck/1 -> Abs/1
  CurrentCheck/1 -> Abs1/1
  Unit Delay/1 -> Logical Operator/3
  Abs/1 -> Compare To Constant/1
  Abs1/1 -> Compare To Constant1/1
  Compare To Constant1/1 -> Logical Operator/1
  Compare To Constant/1 -> Logical Operator/2
  Logical Operator/1 -> ErrorFlag/1, Unit Delay/1

== system EulerPIDJoint_Copy/Controller/PID Controller/PID Controller/Controller Axis 1/PosAdj ==
  Pos : Inport
  Abs : Abs
  Add : Sum  Inputs=+-
  Add1 : Sum  Inputs=+-
  Compare To Constant : simulink/Logic and Bit Operations/Compare To Constant  SystemSampleTime=-1  relop=>=  const=pi/2  LogicOutDataTypeMode=uint8  ZeroCross=off
  Constant : Constant  Value=2*pi  SampleTime=Ts
  Int : DiscreteTransferFcn  Numerator=[1 0]  Denominator=[1 -1]  InitialStates=a1/180*pi  SampleTime=Ts
  Integer Delay : simulink/Discrete/Integer Delay  NumDelays=1  InputProcessing=Inherited  vinit=a1/180*pi  samptime=-1
  Product : Product  RndMeth=Zero
  Product1 : Product  RndMeth=Zero
  Sign : Signum
  PosAdj : Outport
  wires:
  Add1/1 -> Int/1
  Pos/1 -> Add/1, Integer Delay/1
  Int/1 -> PosAdj/1
  Add/1 -> Abs/1, Add1/1, Sign/1
  Integer Delay/1 -> Add/2
  Compare To Constant/1 -> Product/2
  Product/1 -> Add1/2
  Abs/1 -> Compare To Constant/1
  Constant/1 -> Product1/2
  Product1/1 -> Product/1
  Sign/1 -> Product1/1

== system EulerPIDJoint_Copy/Controller/PID Controller/PID Controller/Controller Axis 1/controller: PID ==
  Error : Inport
  Add1 : Sum  Inputs=+++
  D : Gain  Gain=Kd
  Diff : simulink/Discrete/Difference  SystemSampleTime=-1  ICPrevInput=0.0  OutMin=[]  OutMax=[]  OutDataType=sfix(16)  OutScaling=2^-10  DoSatur=off
  I : Gain  Gain=Ki
  Int : DiscreteTransferFcn  Numerator=[1 0]  Denominator=[1 -1]  SampleTime=Ts
  Saturation : Saturate  UpperLimit=LimitSet  LowerLimit=-LimitSet  SampleTime=Ts
      settings: AttributesFormatString=%<UpperLimit>\n%<LowerLimit>
  Saturation1 : Saturate  UpperLimit=LimitSet  LowerLimit=-LimitSet  SampleTime=Ts
      settings: AttributesFormatString=%<UpperLimit>\n%<LowerLimit>
  p : Gain  Gain=Kp
  Ctl : Outport
  wires:
  Error/1 -> p/1, I/1, D/1
  p/1 -> Add1/1
  I/1 -> Int/1
  Add1/1 -> Ctl/1
  D/1 -> Diff/1
  Diff/1 -> Saturation1/1
  Int/1 -> Saturation/1
  Saturation/1 -> Add1/2
  Saturation1/1 -> Add1/3

== system EulerPIDJoint_Copy/Controller/PID Controller/PID Controller/Controller Axis 1/controller: PID1 ==
  Error : Inport
  Add1 : Sum  Inputs=+++
  D : Gain  Gain=Kd
  Diff : simulink/Discrete/Difference  SystemSampleTime=-1  ICPrevInput=0.0  OutMin=[]  OutMax=[]  OutDataType=sfix(16)  OutScaling=2^-10  DoSatur=off
  I : Gain  Gain=Ki
  Int : DiscreteTransferFcn  Numerator=[1 0]  Denominator=[1 -1]  SampleTime=Ts
  Saturation1 : Saturate  UpperLimit=LimitSet  LowerLimit=-LimitSet  SampleTime=Ts
      settings: AttributesFormatString=%<UpperLimit>\n%<LowerLimit>
  Saturation2 : Saturate  UpperLimit=LimitSet  LowerLimit=-LimitSet  SampleTime=Ts
      settings: AttributesFormatString=%<UpperLimit>\n%<LowerLimit>
  p : Gain  Gain=Kp
  Ctl : Outport
  wires:
  Int/1 -> Saturation2/1
  Diff/1 -> Saturation1/1
  D/1 -> Diff/1
  Add1/1 -> Ctl/1
  I/1 -> Int/1
  p/1 -> Add1/1
  Error/1 -> D/1, I/1, p/1
  Saturation2/1 -> Add1/2
  Saturation1/1 -> Add1/3

== system EulerPIDJoint_Copy/Controller/PID Controller/PID Controller/Controller Axis 2/EncDiff2Vel ==
  Enc : Inport
  Add : Sum  Inputs=+-
  Discrete  2nd-Order Filter : powerlib_extras/Discrete  Control Blocks/Discrete  2nd-Order Filter  DialogController=POWERSYS.PowerSysDialog  SystemSampleTime=-1  FilterType=Lowpass  Fo=1000  Zeta=0.707  Ts=Ts  Initialize=off  Vac_Init=[0.8 -25 60]  Vdc_Init=-0.4  PlotResponse=off  param1=[1 5000 10]
  Integer Delay : simulink/Discrete/Integer Delay  NumDelays=1  InputProcessing=Inherited  vinit=a2/180*pi  samptime=-1
  Vel : Outport
  wires:
  Integer Delay/1 -> Add/2
  Enc/1 -> Add/1, Integer Delay/1
  Discrete  2nd-Order Filter/1 -> Vel/1
  Add/1 -> Discrete  2nd-Order Filter/1

== system EulerPIDJoint_Copy/Controller/PID Controller/PID Controller/Controller Axis 2/Error Check and Lock Error ==
  CurrentCheck : Inport
  VelocityCheck : Inport  Port=2
  Abs : Abs
  Abs1 : Abs
  Compare To Constant : simulink/Logic and Bit Operations/Compare To Constant  SystemSampleTime=-1  relop=<=  const=VelErrorCheckLimit  LogicOutDataTypeMode=uint8  ZeroCross=off
  Compare To Constant1 : simulink/Logic and Bit Operations/Compare To Constant  SystemSampleTime=-1  relop=<=  const=VLLimit *1.01  LogicOutDataTypeMode=uint8  ZeroCross=off
  Logical Operator : Logic  Inputs=3  AllPortsSameDT=off  OutDataTypeStr=boolean
  Unit Delay : UnitDelay  X0=1  SampleTime=Ts
  ErrorFlag : Outport
  wires:
  Logical Operator/1 -> Unit Delay/1, ErrorFlag/1
  Compare To Constant/1 -> Logical Operator/2
  Compare To Constant1/1 -> Logical Operator/1
  Abs1/1 -> Compare To Constant1/1
  Abs/1 -> Compare To Constant/1
  Unit Delay/1 -> Logical Operator/3
  CurrentCheck/1 -> Abs1/1
  VelocityCheck/1 -> Abs/1

== system EulerPIDJoint_Copy/Controller/PID Controller/PID Controller/Controller Axis 2/PosAdj ==
  Pos : Inport
  Abs : Abs
  Add : Sum  Inputs=+-
  Add1 : Sum  Inputs=+-
  Compare To Constant : simulink/Logic and Bit Operations/Compare To Constant  SystemSampleTime=-1  relop=>=  const=pi/2  LogicOutDataTypeMode=uint8  ZeroCross=off
  Constant : Constant  Value=2*pi  SampleTime=Ts
  Int : DiscreteTransferFcn  Numerator=[1 0]  Denominator=[1 -1]  InitialStates=a2/180*pi  SampleTime=Ts
  Integer Delay : simulink/Discrete/Integer Delay  NumDelays=1  InputProcessing=Inherited  vinit=a2/180*pi  samptime=-1
  Product : Product  RndMeth=Zero
  Product1 : Product  RndMeth=Zero
  Sign : Signum
  PosAdj : Outport
  wires:
  Add1/1 -> Int/1
  Pos/1 -> Add/1, Integer Delay/1
  Int/1 -> PosAdj/1
  Add/1 -> Abs/1, Add1/1, Sign/1
  Integer Delay/1 -> Add/2
  Compare To Constant/1 -> Product/2
  Product/1 -> Add1/2
  Abs/1 -> Compare To Constant/1
  Constant/1 -> Product1/2
  Product1/1 -> Product/1
  Sign/1 -> Product1/1

== system EulerPIDJoint_Copy/Controller/PID Controller/PID Controller/Controller Axis 2/controller: PID ==
  Error : Inport
  Add1 : Sum  Inputs=+++
  D : Gain  Gain=Kd
  Diff : simulink/Discrete/Difference  SystemSampleTime=-1  ICPrevInput=0.0  OutMin=[]  OutMax=[]  OutDataType=sfix(16)  OutScaling=2^-10  DoSatur=off
  I : Gain  Gain=Ki
  Int : DiscreteTransferFcn  Numerator=[1 0]  Denominator=[1 -1]  SampleTime=Ts
  Saturation : Saturate  UpperLimit=LimitSet  LowerLimit=-LimitSet  SampleTime=Ts
      settings: AttributesFormatString=%<UpperLimit>\n%<LowerLimit>
  Saturation1 : Saturate  UpperLimit=LimitSet  LowerLimit=-LimitSet  SampleTime=Ts
      settings: AttributesFormatString=%<UpperLimit>\n%<LowerLimit>
  p : Gain  Gain=Kp
  Ctl : Outport
  wires:
  Saturation1/1 -> Add1/3
  Saturation/1 -> Add1/2
  Int/1 -> Saturation/1
  Diff/1 -> Saturation1/1
  D/1 -> Diff/1
  Add1/1 -> Ctl/1
  I/1 -> Int/1
  p/1 -> Add1/1
  Error/1 -> D/1, I/1, p/1

== system EulerPIDJoint_Copy/Controller/PID Controller/PID Controller/Controller Axis 2/controller: PID1 ==
  Error : Inport
  Add1 : Sum  Inputs=+++
  D : Gain  Gain=Kd
  Diff : simulink/Discrete/Difference  SystemSampleTime=-1  ICPrevInput=0.0  OutMin=[]  OutMax=[]  OutDataType=sfix(16)  OutScaling=2^-10  DoSatur=off
  I : Gain  Gain=Ki
  Int : DiscreteTransferFcn  Numerator=[1 0]  Denominator=[1 -1]  SampleTime=Ts
  Saturation1 : Saturate  UpperLimit=LimitSet  LowerLimit=-LimitSet  SampleTime=Ts
      settings: AttributesFormatString=%<UpperLimit>\n%<LowerLimit>
  Saturation2 : Saturate  UpperLimit=LimitSet  LowerLimit=-LimitSet  SampleTime=Ts
      settings: AttributesFormatString=%<UpperLimit>\n%<LowerLimit>
  p : Gain  Gain=Kp
  Ctl : Outport
  wires:
  Saturation1/1 -> Add1/3
  Saturation2/1 -> Add1/2
  Error/1 -> p/1, I/1, D/1
  p/1 -> Add1/1
  I/1 -> Int/1
  Add1/1 -> Ctl/1
  D/1 -> Diff/1
  Diff/1 -> Saturation1/1
  Int/1 -> Saturation2/1

== system EulerPIDJoint_Copy/Controller/PID Controller/PID Controller/Controller Axis 3/EncDiff2Vel ==
  Enc : Inport
  Add : Sum  Inputs=+-
  Discrete  2nd-Order Filter : powerlib_extras/Discrete  Control Blocks/Discrete  2nd-Order Filter  DialogController=POWERSYS.PowerSysDialog  SystemSampleTime=-1  FilterType=Lowpass  Fo=1000  Zeta=0.707  Ts=Ts  Initialize=off  Vac_Init=[0.8 -25 60]  Vdc_Init=-0.4  PlotResponse=off  param1=[1 5000 10]
  Integer Delay : simulink/Discrete/Integer Delay  NumDelays=1  InputProcessing=Inherited  vinit=a3/180*pi  samptime=-1
  Vel : Outport
  wires:
  Add/1 -> Discrete  2nd-Order Filter/1
  Discrete  2nd-Order Filter/1 -> Vel/1
  Enc/1 -> Integer Delay/1, Add/1
  Integer Delay/1 -> Add/2

== system EulerPIDJoint_Copy/Controller/PID Controller/PID Controller/Controller Axis 3/Error Check and Lock Error ==
  CurrentCheck : Inport
  VelocityCheck : Inport  Port=2
  Abs : Abs
  Abs1 : Abs
  Compare To Constant : simulink/Logic and Bit Operations/Compare To Constant  SystemSampleTime=-1  relop=<=  const=VelErrorCheckLimit  LogicOutDataTypeMode=uint8  ZeroCross=off
  Compare To Constant1 : simulink/Logic and Bit Operations/Compare To Constant  SystemSampleTime=-1  relop=<=  const=VLLimit *1.01  LogicOutDataTypeMode=uint8  ZeroCross=off
  Logical Operator : Logic  Inputs=3  AllPortsSameDT=off  OutDataTypeStr=boolean
  Unit Delay : UnitDelay  X0=1  SampleTime=Ts
  ErrorFlag : Outport
  wires:
  VelocityCheck/1 -> Abs/1
  CurrentCheck/1 -> Abs1/1
  Unit Delay/1 -> Logical Operator/3
  Abs/1 -> Compare To Constant/1
  Abs1/1 -> Compare To Constant1/1
  Compare To Constant1/1 -> Logical Operator/1
  Compare To Constant/1 -> Logical Operator/2
  Logical Operator/1 -> ErrorFlag/1, Unit Delay/1

== system EulerPIDJoint_Copy/Controller/PID Controller/PID Controller/Controller Axis 3/PosAdj ==
  Pos : Inport
  Abs : Abs
  Add : Sum  Inputs=+-
  Add1 : Sum  Inputs=+-
  Compare To Constant : simulink/Logic and Bit Operations/Compare To Constant  SystemSampleTime=-1  relop=>=  const=pi/2  LogicOutDataTypeMode=uint8  ZeroCross=off
  Constant : Constant  Value=2*pi  SampleTime=Ts
  Int : DiscreteTransferFcn  Numerator=[1 0]  Denominator=[1 -1]  InitialStates=a3/180*pi  SampleTime=Ts
  Integer Delay : simulink/Discrete/Integer Delay  NumDelays=1  InputProcessing=Inherited  vinit=a3/180*pi  samptime=-1
  Product : Product  RndMeth=Zero
  Product1 : Product  RndMeth=Zero
  Sign : Signum
  PosAdj : Outport
  wires:
  Add1/1 -> Int/1
  Pos/1 -> Add/1, Integer Delay/1
  Int/1 -> PosAdj/1
  Add/1 -> Abs/1, Add1/1, Sign/1
  Integer Delay/1 -> Add/2
  Compare To Constant/1 -> Product/2
  Product/1 -> Add1/2
  Abs/1 -> Compare To Constant/1
  Constant/1 -> Product1/2
  Product1/1 -> Product/1
  Sign/1 -> Product1/1

== system EulerPIDJoint_Copy/Controller/PID Controller/PID Controller/Controller Axis 3/controller: PID ==
  Error : Inport
  Add1 : Sum  Inputs=+++
  D : Gain  Gain=Kd
  Diff : simulink/Discrete/Difference  SystemSampleTime=-1  ICPrevInput=0.0  OutMin=[]  OutMax=[]  OutDataType=sfix(16)  OutScaling=2^-10  DoSatur=off
  I : Gain  Gain=Ki
  Int : DiscreteTransferFcn  Numerator=[1 0]  Denominator=[1 -1]  SampleTime=Ts
  Saturation : Saturate  UpperLimit=LimitSet  LowerLimit=-LimitSet  SampleTime=Ts
      settings: AttributesFormatString=%<UpperLimit>\n%<LowerLimit>
  Saturation1 : Saturate  UpperLimit=LimitSet  LowerLimit=-LimitSet  SampleTime=Ts
      settings: AttributesFormatString=%<UpperLimit>\n%<LowerLimit>
  p : Gain  Gain=Kp
  Ctl : Outport
  wires:
  Error/1 -> p/1, I/1, D/1
  p/1 -> Add1/1
  I/1 -> Int/1
  Add1/1 -> Ctl/1
  D/1 -> Diff/1
  Diff/1 -> Saturation1/1
  Int/1 -> Saturation/1
  Saturation/1 -> Add1/2
  Saturation1/1 -> Add1/3

== system EulerPIDJoint_Copy/Controller/PID Controller/PID Controller/Controller Axis 3/controller: PID1 ==
  Error : Inport
  Add1 : Sum  Inputs=+++
  D : Gain  Gain=Kd
  Diff : simulink/Discrete/Difference  SystemSampleTime=-1  ICPrevInput=0.0  OutMin=[]  OutMax=[]  OutDataType=sfix(16)  OutScaling=2^-10  DoSatur=off
  I : Gain  Gain=Ki
  Int : DiscreteTransferFcn  Numerator=[1 0]  Denominator=[1 -1]  SampleTime=Ts
  Saturation1 : Saturate  UpperLimit=LimitSet  LowerLimit=-LimitSet  SampleTime=Ts
      settings: AttributesFormatString=%<UpperLimit>\n%<LowerLimit>
  Saturation2 : Saturate  UpperLimit=LimitSet  LowerLimit=-LimitSet  SampleTime=Ts
      settings: AttributesFormatString=%<UpperLimit>\n%<LowerLimit>
  p : Gain  Gain=Kp
  Ctl : Outport
  wires:
  Int/1 -> Saturation2/1
  Diff/1 -> Saturation1/1
  D/1 -> Diff/1
  Add1/1 -> Ctl/1
  I/1 -> Int/1
  p/1 -> Add1/1
  Error/1 -> D/1, I/1, p/1
  Saturation2/1 -> Add1/2
  Saturation1/1 -> Add1/3

== system EulerPIDJoint_Copy/Controller/PID Controller/PID Controller/Controller Axis 4/EncDiff2Vel ==
  Enc : Inport
  Add : Sum  Inputs=+-
  Discrete  2nd-Order Filter : powerlib_extras/Discrete  Control Blocks/Discrete  2nd-Order Filter  DialogController=POWERSYS.PowerSysDialog  SystemSampleTime=-1  FilterType=Lowpass  Fo=1000  Zeta=0.707  Ts=Ts  Initialize=off  Vac_Init=[0.8 -25 60]  Vdc_Init=-0.4  PlotResponse=off  param1=[1 5000 10]
  Integer Delay : simulink/Discrete/Integer Delay  NumDelays=1  InputProcessing=Inherited  vinit=a4/180*pi  samptime=-1
  Vel : Outport
  wires:
  Integer Delay/1 -> Add/2
  Enc/1 -> Add/1, Integer Delay/1
  Discrete  2nd-Order Filter/1 -> Vel/1
  Add/1 -> Discrete  2nd-Order Filter/1

== system EulerPIDJoint_Copy/Controller/PID Controller/PID Controller/Controller Axis 4/Error Check and Lock Error ==
  CurrentCheck : Inport
  VelocityCheck : Inport  Port=2
  Abs : Abs
  Abs1 : Abs
  Compare To Constant : simulink/Logic and Bit Operations/Compare To Constant  SystemSampleTime=-1  relop=<=  const=VelErrorCheckLimit  LogicOutDataTypeMode=uint8  ZeroCross=off
  Compare To Constant1 : simulink/Logic and Bit Operations/Compare To Constant  SystemSampleTime=-1  relop=<=  const=VLLimit *1.01  LogicOutDataTypeMode=uint8  ZeroCross=off
  Logical Operator : Logic  Inputs=3  AllPortsSameDT=off  OutDataTypeStr=boolean
  Unit Delay : UnitDelay  X0=1  SampleTime=Ts
  ErrorFlag : Outport
  wires:
  Logical Operator/1 -> Unit Delay/1, ErrorFlag/1
  Compare To Constant/1 -> Logical Operator/2
  Compare To Constant1/1 -> Logical Operator/1
  Abs1/1 -> Compare To Constant1/1
  Abs/1 -> Compare To Constant/1
  Unit Delay/1 -> Logical Operator/3
  CurrentCheck/1 -> Abs1/1
  VelocityCheck/1 -> Abs/1

== system EulerPIDJoint_Copy/Controller/PID Controller/PID Controller/Controller Axis 4/PosAdj ==
  Pos : Inport
  Abs : Abs
  Add : Sum  Inputs=+-
  Add1 : Sum  Inputs=+-
  Compare To Constant : simulink/Logic and Bit Operations/Compare To Constant  SystemSampleTime=-1  relop=>=  const=pi/2  LogicOutDataTypeMode=uint8  ZeroCross=off
  Constant : Constant  Value=2*pi  SampleTime=Ts
  Int : DiscreteTransferFcn  Numerator=[1 0]  Denominator=[1 -1]  SampleTime=Ts
  Integer Delay : simulink/Discrete/Integer Delay  NumDelays=1  InputProcessing=Inherited  vinit=a4/180*pi  samptime=-1
  Product : Product  RndMeth=Zero
  Product1 : Product  RndMeth=Zero
  Sign : Signum
  PosAdj : Outport
  wires:
  Add1/1 -> Int/1
  Pos/1 -> Add/1, Integer Delay/1
  Int/1 -> PosAdj/1
  Add/1 -> Abs/1, Add1/1, Sign/1
  Integer Delay/1 -> Add/2
  Compare To Constant/1 -> Product/2
  Product/1 -> Add1/2
  Abs/1 -> Compare To Constant/1
  Constant/1 -> Product1/2
  Product1/1 -> Product/1
  Sign/1 -> Product1/1
